simulink model "ITCG_PNG_3D_salvo_simulation2"  (R2023b)
settings: Solver=ode4  StartTime=0.0  StopTime=30  FixedStep=1/10  RelTol=1e-3
libraries: simulink x4, simulink_extras x4
(part 1 of 2)
settings Model: NumberOfSteps=10  PacingRate=5  Creator=Administrator  LastModifiedBy=Administrator
settings DebuggingCC: UnderSpecifiedDimensionMsg=warning

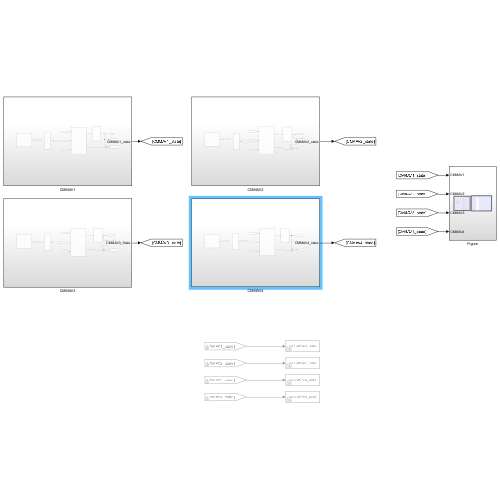
[thumbnail: Simulink's stored preview of the top-level diagram]
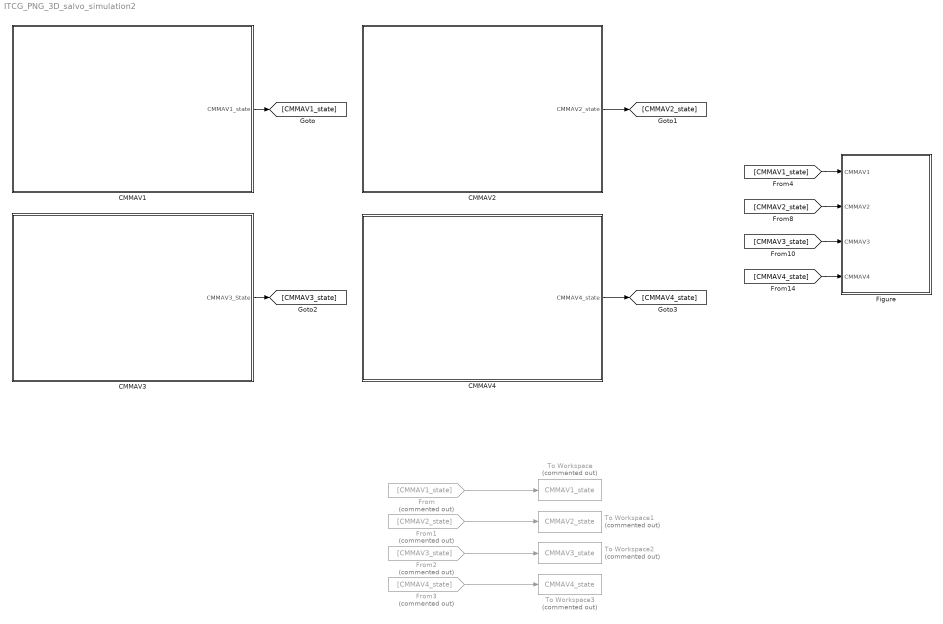
== system ITCG_PNG_3D_salvo_simulation2 ==
  CMMAV1 : Subsystem
  CMMAV2 : Subsystem
  CMMAV3 : Subsystem
  CMMAV4 : Subsystem
  Figure : Subsystem
  From : From  Commented=on  GotoTag=CMMAV1_state
  From1 : From  Commented=on  GotoTag=CMMAV2_state
  From2 : From  Commented=on  GotoTag=CMMAV3_state
  From3 : From  Commented=on  GotoTag=CMMAV4_state
  To Workspace : ToWorkspace  Commented=on  VariableName=CMMAV1_state  SaveFormat=Timeseries  SampleTime=-1
  To Workspace1 : ToWorkspace  Commented=on  VariableName=CMMAV2_state  SaveFormat=Timeseries  SampleTime=-1
  To Workspace2 : ToWorkspace  Commented=on  VariableName=CMMAV3_state  SaveFormat=Timeseries  SampleTime=-1
  To Workspace3 : ToWorkspace  Commented=on  VariableName=CMMAV4_state  SaveFormat=Timeseries  SampleTime=-1
  wires:
  CMMAV1/1(CMMAV1_state) -> [CMMAV1_state]
  CMMAV2/1(CMMAV2_state) -> [CMMAV2_state]
  CMMAV3/1(CMMAV3_State) -> [CMMAV3_state]
  CMMAV4/1(CMMAV4_state) -> [CMMAV4_state]
  From/1 -> To Workspace/1
  From1/1 -> To Workspace1/1
  From2/1 -> To Workspace2/1
  From3/1 -> To Workspace3/1
  [CMMAV2_state] -> Figure/2(CMMAV2)
  [CMMAV1_state] -> Figure/1(CMMAV1)
  [CMMAV3_state] -> Figure/3(CMMAV3)
  [CMMAV4_state] -> Figure/4(CMMAV4)

== system ITCG_PNG_3D_salvo_simulation2/CMMAV1 ==
  Guidance : Subsystem
  Mux : Mux  Inputs=2
  Parameter init : Subsystem
  Point Mass Model : Subsystem
  Target : Subsystem  TreatAsAtomicUnit=on
  To File : ToFile  Filename=CMMAV1_ITCG_PNG.mat
  CMMAV1_state : Outport
  wires:
  [Parameter] -> Guidance/3(Parameter)
  [Taregt_info] -> Guidance/2(Target_info)
  [CMMAV1_state] -> Guidance/1(CMMAV1_state)
  Guidance/1(CMMAV1_input) -> Point Mass Model/1(CMMAV1_input)
  Parameter init/1(Parameter) -> [Parameter]
  Guidance/2(CMMAV1_param) -> Mux/2
  Mux/1 -> To File/1
  Point Mass Model/1(CMMAV1_state) -> [CMMAV1_state], Mux/1, CMMAV1_state/1
  Target/1(Target_info) -> [Taregt_info]

== system ITCG_PNG_3D_salvo_simulation2/CMMAV2 ==
  CMMAV2 : Subsystem
  Guidance : Subsystem
  Mux : Mux  Inputs=2
  Parameter init : Subsystem
  Target : Subsystem  TreatAsAtomicUnit=on
  To File : ToFile  Filename=CMMAV2_ITCG_PNG.mat
  CMMAV2_state : Outport
  wires:
  [Parameter] -> Guidance/3(Parameter)
  Guidance/1(CMMAV2_input) -> CMMAV2/1(CMMAV2_input)
  [CMMAV2_state] -> Guidance/1(CMMAV2_state)
  Parameter init/1(Parameter) -> [Parameter]
  [Taregt_info] -> Guidance/2(Target_info)
  Guidance/2(CMMAV2_param) -> Mux/2
  Mux/1 -> To File/1
  CMMAV2/1(CMMAV2_state) -> [CMMAV2_state], Mux/1, CMMAV2_state/1
  Target/1(Target_info) -> [Taregt_info]

== system ITCG_PNG_3D_salvo_simulation2/CMMAV3 ==
  CMMAV3 : Subsystem
  Guidance : Subsystem
  Mux : Mux  Inputs=2
  Parameter init : Subsystem
  Target : Subsystem  TreatAsAtomicUnit=on
  To File : ToFile  Filename=CMMAV3_ITCG_PNG.mat
  CMMAV3_State : Outport
  wires:
  [Taregt_info] -> Guidance/2(Target_info)
  [Parameter] -> Guidance/3(Parameter)
  Parameter init/1(Parameter) -> [Parameter]
  Guidance/1(CMMAV3_input) -> CMMAV3/1(CMMAV3_input)
  [CMMAV3_state] -> Guidance/1(CMMAV3_state)
  Guidance/2(CMMAV1_param) -> Mux/2
  Mux/1 -> To File/1
  CMMAV3/1(CMMAV3_state) -> [CMMAV3_state], Mux/1, CMMAV3_State/1
  Target/1(Target_info) -> [Taregt_info]

== system ITCG_PNG_3D_salvo_simulation2/CMMAV4 ==
  CMMAV4 : Subsystem
  Guidance : Subsystem
  Mux : Mux  Inputs=2
  Parameter init : Subsystem
  Target : Subsystem  TreatAsAtomicUnit=on
  To File : ToFile  Filename=CMMAV4_ITCG_PNG.mat
  CMMAV4_state : Outport
  wires:
  [Taregt_info] -> Guidance/2(Target_info)
  Guidance/1(CMMAV4_input) -> CMMAV4/1(CMMAV4_input)
  [CMMAV4_state] -> Guidance/1(CMMAV4_state)
  [Parameter] -> Guidance/3(Parameter)
  Parameter init/1(Parameter) -> [Parameter]
  CMMAV4/1(CMMAV4_state) -> [CMMAV4_state], Mux/1, CMMAV4_state/1
  Mux/1 -> To File/1
  Guidance/2(CMMAV1_param) -> Mux/2
  Target/1(Target_info) -> [Taregt_info]

== system ITCG_PNG_3D_salvo_simulation2/Figure ==
  note: Figure
  note: Input parameter
  CMMAV1 : Inport
  CMMAV2 : Inport  Port=2
  CMMAV3 : Inport  Port=3
  CMMAV4 : Inport  Port=4
  Bus Selector{,1..3} (4 alike) : BusSelector  OutputSignals=Pos_M_m
  Demux{,1..3} (4 alike) : Demux  Outputs=3
  MATLAB Function : MATLAB Function  TreatAsAtomicUnit=on
  wires:
  Demux/2 -> [CMMAV1_y]
  Demux/1 -> [CMMAV1_x]
  Demux/3 -> [CMMAV1_z]
  [CMMAV1] -> Demux/1
  CMMAV1/1 -> Bus Selector/1
  CMMAV2/1 -> Bus Selector1/1
  CMMAV3/1 -> Bus Selector2/1
  CMMAV4/1 -> Bus Selector3/1
  Bus Selector/1 -> [CMMAV1]  "<Pos_M_m>"
  Bus Selector1/1 -> [CMMAV2]  "<Pos_M_m>"
  Bus Selector2/1 -> [CMMAV3]  "<Pos_M_m>"
  Bus Selector3/1 -> [CMMAV4]  "<Pos_M_m>"
  Demux1/1 -> [CMMAV2_x]
  Demux1/3 -> [CMMAV2_z]
  Demux1/2 -> [CMMAV2_y]
  [CMMAV2] -> Demux1/1
  Demux2/2 -> [CMMAV3_y]
  Demux2/1 -> [CMMAV3_x]
  Demux2/3 -> [CMMAV3_z]
  [CMMAV3] -> Demux2/1
  Demux3/2 -> [CMMAV4_y]
  Demux3/1 -> [CMMAV4_x]
  Demux3/3 -> [CMMAV4_z]
  [CMMAV4] -> Demux3/1
  [CMMAV1_x] -> MATLAB Function/1(CMMAV1_x)
  [CMMAV1_y] -> MATLAB Function/2(CMMAV1_y)
  [CMMAV1_z] -> MATLAB Function/3(CMMAV1_z)
  [CMMAV2_x] -> MATLAB Function/4(CMMAV2_x)
  [CMMAV2_y] -> MATLAB Function/5(CMMAV2_y)
  [CMMAV2_z] -> MATLAB Function/6(CMMAV2_z)
  [CMMAV3_x] -> MATLAB Function/7(CMMAV3_x)
  [CMMAV3_y] -> MATLAB Function/8(CMMAV3_y)
  [CMMAV3_z] -> MATLAB Function/9(CMMAV3_z)
  [CMMAV4_x] -> MATLAB Function/10(CMMAV4_x)
  [CMMAV4_y] -> MATLAB Function/11(CMMAV4_y)
  [CMMAV4_z] -> MATLAB Function/12(CMMAV4_z)

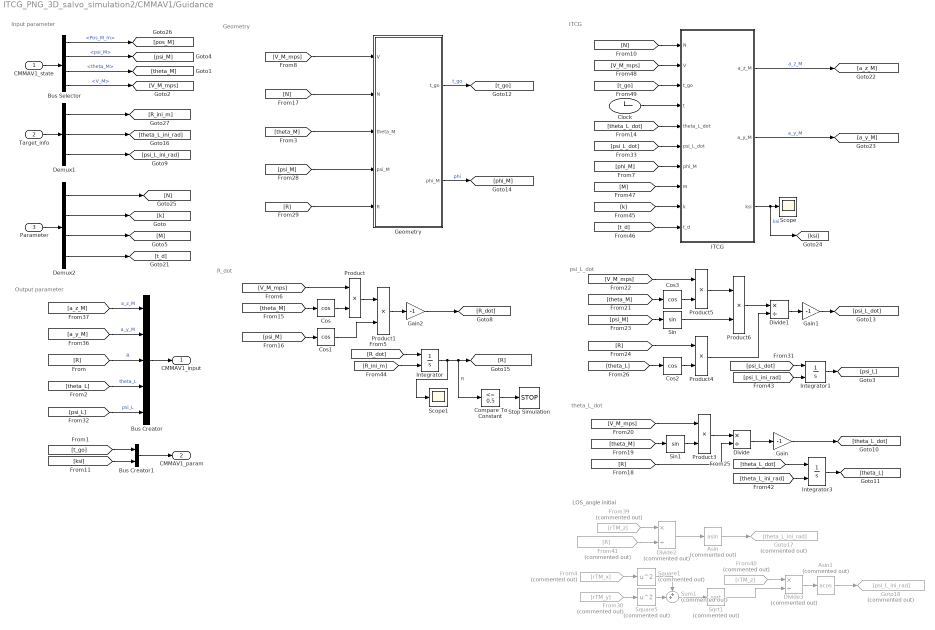
== system ITCG_PNG_3D_salvo_simulation2/CMMAV1/Guidance ==
  note: Input parameter
  note: ITCG
  note: R_dot
  note: psi_L_dot
  note: theta_L_dot
  note: LOS_angle initial
  note: Output parameter
  note: Geometry
  CMMAV1_state : Inport
  Target_info : Inport  Port=2
  Parameter : Inport  Port=3
  Asin : Trigonometry  Commented=on  Operator=asin
  Asin1 : Trigonometry  Commented=on  Operator=acos
  Bus Creator : BusCreator  Inputs=5
  Bus Creator1 : BusCreator  Inputs=2
  Bus Selector : BusSelector  OutputSignals=Pos_M_m,psi_M,theta_M,V_M
  Clock : Clock
  Compare To Constant : simulink/Logic and Bit Operations/Compare To Constant  relop=<=  const=0.5  OutDataTypeStr=boolean
  Cos{,1..3} (4 alike) : Trigonometry  Operator=cos
  Demux1 : Demux  Outputs=3
  Demux2 : Demux
  Divide : Product  Inputs=*/
  Divide1 : Product  Inputs=*/
  Divide2 : Product  Commented=on  Inputs=*/
  Divide3 : Product  Commented=on  Inputs=*/
  From30 : From  Commented=on  GotoTag=rTM_y
  From39 : From  Commented=on  GotoTag=rTM_z
  From4 : From  Commented=on  GotoTag=rTM_x
  From40 : From  Commented=on  GotoTag=rTM_z
  From41 : From  Commented=on  GotoTag=R
  Gain : Gain  Gain=-1
  Gain1 : Gain  Gain=-1
  Gain2 : Gain  Gain=-1
  Geometry : MATLAB Function  TreatAsAtomicUnit=on
  Goto17 : Goto  Commented=on  GotoTag=theta_L_ini_rad
  Goto18 : Goto  Commented=on  GotoTag=psi_L_ini_rad
  ITCG : MATLAB Function  TreatAsAtomicUnit=on
  Integrator : Integrator  InitialConditionSource=external  InitialCondition=sqrt(300^2+500^2+200^2)
  Integrator1 : Integrator  InitialConditionSource=external
  Integrator3 : Integrator  InitialConditionSource=external
  Product{,1,3..6} (6 alike) : Product
  Scope : Scope
  Scope1 : Scope
  Sin : Trigonometry
  Sin1 : Trigonometry
  Sqrt1 : Sqrt  Commented=on
  Square1 : Math  Commented=on  Operator=square
  Square5 : Math  Commented=on  Operator=square
  Stop Simulation : Stop
  Sum1 : Sum  Commented=on  Inputs=++|
  CMMAV1_input : Outport
  CMMAV1_param : Outport  Port=2
  wires:
  Product1/1 -> Gain2/1
  Gain2/1 -> [R_dot]
  [theta_L] -> Cos2/1
  [theta_L_dot] -> Integrator3/1
  Gain/1 -> [theta_L_dot]
  Product5/1 -> Product6/1
  Divide1/1 -> Gain1/1
  [V_M_mps] -> Product3/1
  [V_M_mps] -> Product5/1
  [theta_M] -> Sin1/1
  [R] -> Divide/2
  [theta_M] -> Cos3/1
  Divide/1 -> Gain/1
  [theta_M] -> Cos/1
  [R] -> Product4/1
  Product4/1 -> Divide1/2
  Integrator3/1 -> [theta_L]
  [psi_L_dot] -> Integrator1/1
  Sin1/1 -> Product3/2
  Product3/1 -> Divide/1
  [psi_M] -> Cos1/1
  Cos/1 -> Product/2
  Integrator1/1 -> [psi_L]
  Product6/1 -> Divide1/1
  [psi_M] -> Sin/1
  Compare To Constant/1 -> Stop Simulation/1
  [V_M_mps] -> Product/1
  Cos3/1 -> Product5/2
  Sin/1 -> Product6/2
  Integrator/1 -> Scope1/1, [R], Compare To Constant/1  "R"
  Product/1 -> Product1/1
  Cos2/1 -> Product4/2
  Cos1/1 -> Product1/2
  Gain1/1 -> [psi_L_dot]
  [R_dot] -> Integrator/1
  Divide3/1 -> Asin1/1
  Sum1/1 -> Sqrt1/1
  From30/1 -> Square5/1
  Square5/1 -> Sum1/2
  Square1/1 -> Sum1/1
  Asin/1 -> Goto17/1
  Sqrt1/1 -> Divide3/2
  From41/1 -> Divide2/2
  Asin1/1 -> Goto18/1
  From40/1 -> Divide3/1
  From39/1 -> Divide2/1
  From4/1 -> Square1/1
  Divide2/1 -> Asin/1
  CMMAV1_state/1 -> Bus Selector/1
  Target_info/1 -> Demux1/1
  Demux2/1 -> [N]
  Parameter/1 -> Demux2/1
  Bus Selector/1 -> [pos_M]  "<Pos_M_m>"
  Bus Selector/4 -> [V_M_mps]  "<V_M>"
  Demux1/2 -> [theta_L_ini_rad]
  Demux1/3 -> [psi_L_ini_rad]
  Demux1/1 -> [R_ini_m]
  [psi_L] -> Bus Creator/5  "psi_L"
  [theta_L] -> Bus Creator/4  "theta_L"
  Bus Creator/1 -> CMMAV1_input/1
  [a_y_M] -> Bus Creator/2  "a_y_M"
  [R] -> Bus Creator/3  "R"
  [a_z_M] -> Bus Creator/1  "a_z_M"
  [theta_L_ini_rad] -> Integrator3/2
  [psi_L_ini_rad] -> Integrator1/2
  [R_ini_m] -> Integrator/2
  Bus Selector/2 -> [psi_M]  "<psi_M>"
  Bus Selector/3 -> [theta_M]  "<theta_M>"
  Geometry/1(t_go) -> [t_go]  "t_go"
  [psi_M] -> Geometry/4(psi_M)
  Geometry/2(phi_M) -> [phi_M]  "phi"
  [V_M_mps] -> Geometry/1(V)
  [theta_M] -> Geometry/3(theta_M)
  [R] -> Geometry/5(R)
  [N] -> Geometry/2(N)
  [psi_L_dot] -> ITCG/6(psi_L_dot)
  Clock/1 -> ITCG/4(t)
  [t_go] -> ITCG/3(t_go)
  [N] -> ITCG/1(N)
  [M] -> ITCG/8(M)
  [k] -> ITCG/9(k)
  [t_d] -> ITCG/10(t_d)
  [phi_M] -> ITCG/7(phi_M)
  [theta_L_dot] -> ITCG/5(theta_L_dot)
  [V_M_mps] -> ITCG/2(V)
  Demux2/2 -> [k]
  Demux2/3 -> [M]
  Demux2/4 -> [t_d]
  ITCG/1(a_z_M) -> [a_z_M]  "a_z_M"
  ITCG/2(a_y_M) -> [a_y_M]  "a_y_M"
  ITCG/3(ksi) -> [ksi], Scope/1  "ksi"
  [t_go] -> Bus Creator1/1
  [ksi] -> Bus Creator1/2
  Bus Creator1/1 -> CMMAV1_param/1

== system ITCG_PNG_3D_salvo_simulation2/CMMAV1/Parameter init ==
  Constant : Constant  Value=3
  Constant1 : Constant  Value=2
  Constant2 : Constant  Value=10
  Constant3 : Constant  Value=30
  Mux : Mux
  Parameter : Outport
  wires:
  Mux/1 -> Parameter/1
  Constant3/1 -> Mux/4
  Constant2/1 -> Mux/3
  Constant1/1 -> Mux/2
  Constant/1 -> Mux/1

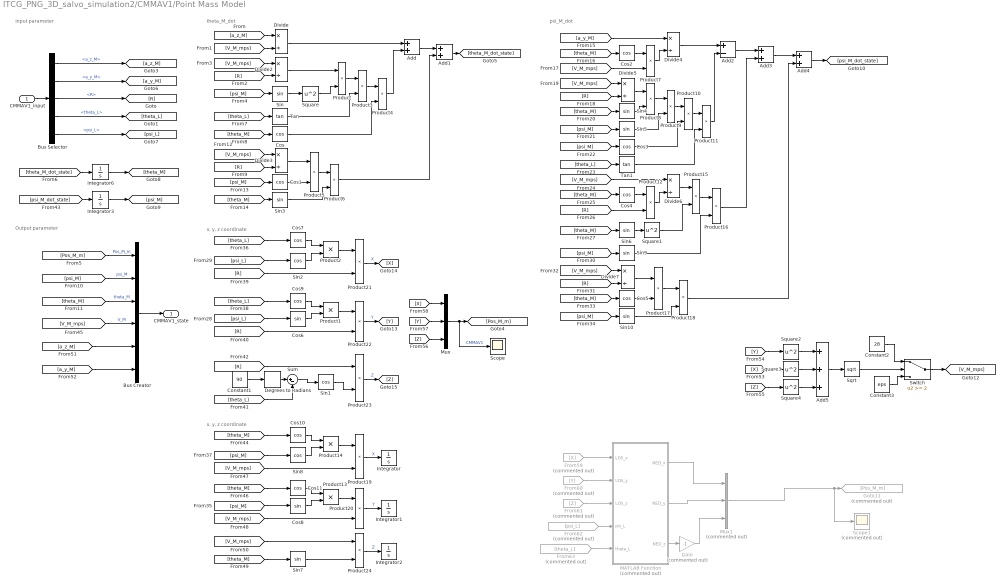
== system ITCG_PNG_3D_salvo_simulation2/CMMAV1/Point Mass Model ==
  note: Input parameter
  note: x, y, z coordinate
  note: theta_M_dot
  note: Output parameter
  note: psi_M_dot
  note: x, y, z coordinate
  CMMAV1_input : Inport
  Add{,1,3..4} (4 alike) : Sum
  Add2 : Sum  Inputs=+-
  Add5 : Sum  Inputs=+++
  Bus Creator : BusCreator  Inputs=6
  Bus Selector : BusSelector  OutputSignals=a_z_M,a_y_M,R,theta_L,psi_L
  Constant1 : Constant  Value=90
  Constant2 : Constant  Value=28
  Constant3 : Constant  Value=eps
  Cos{,1..5,7,9..11} (10 alike) : Trigonometry  Operator=cos
  Cos6 : Trigonometry
  Cos8 : Trigonometry
  Degrees to Radians : simulink_extras/Transformations/Degrees to Radians
  Divide{,2..7} (7 alike) : Product  Inputs=*/
  From59 : From  Commented=on  GotoTag=X
  From60 : From  Commented=on  GotoTag=Y
  From61 : From  Commented=on  GotoTag=Z
  From62 : From  Commented=on  GotoTag=psi_L
  From63 : From  Commented=on  GotoTag=theta_L
  Gain : Gain  Commented=on  Gain=-1
  Goto11 : Goto  Commented=on  GotoTag=Pos_M_m
  Integrator : Integrator
  Integrator1 : Integrator
  Integrator2 : Integrator
  Integrator3 : Integrator  InitialCondition=10*pi/180
  Integrator6 : Integrator  InitialCondition=10*pi/180
  MATLAB Function : MATLAB Function  Commented=on  TreatAsAtomicUnit=on
  Mux : Mux  Inputs=3
  Mux1 : Mux  Commented=on  Inputs=3
  Product{,1..24} (25 alike) : Product
  Scope : Scope
  Scope1 : Scope  Commented=on
  Sin{,3..7,9..10} (8 alike) : Trigonometry
  Sin1 : Trigonometry  Operator=cos
  Sin2 : Trigonometry  Operator=cos
  Sin8 : Trigonometry  Operator=cos
  Sqrt : Sqrt
  Square{,1..4} (5 alike) : Math  Operator=square
  Sum : Sum  Inputs=|+-
  Switch : Switch  Threshold=2  SaturateOnIntegerOverflow=off  InputSameDT=off
  Tan : Trigonometry  Operator=tan
  Tan1 : Trigonometry  Operator=tan
  CMMAV1_state : Outport
  wires:
  [theta_L] -> Tan1/1
  Product16/1 -> Add3/2
  Product9/1 -> Product10/1
  [psi_M] -> Bus Creator/2  "psi_M"
  Tan/1 -> Product3/2
  [psi_M_dot_state] -> Integrator3/1
  [psi_M] -> Sin9/1
  [theta_M] -> Cos/1
  Sin10/1 -> Product18/2
  [psi_M] -> Sin5/1
  Product17/1 -> Product18/1
  [psi_M] -> Sin10/1
  [theta_L] -> Cos9/1
  [V_M_mps] -> Divide/2
  Sin6/1 -> Square1/1
  Product15/1 -> Product16/1
  [V_M_mps] -> Bus Creator/4  "V_M"
  Cos5/1 -> Product17/2
  Sin/1 -> Square/1
  Add2/1 -> Add3/1
  Divide7/1 -> Product17/1
  [theta_M] -> Sin6/1
  [R] -> Divide7/2
  Sin3/1 -> Product6/2
  Add1/1 -> [theta_M_dot_state]
  Sin9/1 -> Product16/2
  Divide6/1 -> Product15/1
  Square1/1 -> Product15/2
  [R] -> Divide3/2
  [a_z_M] -> Divide/1
  [theta_M] -> Cos5/1
  Add3/1 -> Add4/1
  Product12/1 -> Divide6/2
  Product8/1 -> Product9/1
  [a_y_M] -> Divide4/1
  [psi_M] -> Cos3/1
  Product10/1 -> Product11/1
  Product3/1 -> Product4/1
  Divide4/1 -> Add2/1
  Cos3/1 -> Product10/2
  Product11/1 -> Add2/2
  [R] -> Product12/2
  [V_M_mps] -> Divide5/1
  Cos/1 -> Product4/2
  Product5/1 -> Product6/1
  Product6/1 -> Add1/2
  Divide3/1 -> Product5/1
  Cos1/1 -> Product5/2
  Square/1 -> Product/2
  [psi_M] -> Cos1/1
  [V_M_mps] -> Product7/2
  [R] -> Divide2/2
  Cos6/1 -> Product1/2
  [V_M_mps] -> Divide2/1
  [psi_M] -> Sin/1
  Bus Selector/2 -> [a_y_M]  "<a_y_M>"
  [theta_M] -> Sin4/1
  Tan1/1 -> Product11/2
  Integrator6/1 -> [theta_M]
  [theta_M] -> Sin3/1
  [psi_L] -> Cos6/1
  Add/1 -> Add1/1
  Bus Selector/5 -> [psi_L]  "<psi_L>"
  [R] -> Divide5/2
  Product21/1 -> [X]  "X"
  [V_M_mps] -> Divide6/1
  Product1/1 -> Product22/1
  Integrator3/1 -> [psi_M]
  Product/1 -> Product3/1
  Sin2/1 -> Product2/2
  Bus Selector/1 -> [a_z_M]  "<a_z_M>"
  Add4/1 -> [psi_M_dot_state]
  [V_M_mps] -> Divide7/1
  Cos2/1 -> Product7/1
  Mux/1 -> [Pos_M_m], Scope/1  "CMMAV1"
  Bus Selector/3 -> [R]  "<R>"
  [theta_M] -> Bus Creator/3  "theta_M"
  [psi_L] -> Sin2/1
  Divide2/1 -> Product/1
  [theta_M] -> Cos2/1
  Sin4/1 -> Product8/2
  [theta_L] -> Tan/1
  Cos4/1 -> Product12/1
  Product2/1 -> Product21/1
  [theta_M] -> Cos4/1
  Cos9/1 -> Product1/1
  [V_M_mps] -> Divide3/1
  Sin5/1 -> Product9/2
  [theta_L] -> Cos7/1
  Product4/1 -> Add/2
  Product18/1 -> Add4/2
  Product7/1 -> Divide4/2
  Divide5/1 -> Product8/1
  Divide/1 -> Add/1
  Cos7/1 -> Product2/1
  [theta_M_dot_state] -> Integrator6/1
  Product22/1 -> [Y]  "Y"
  [V_M_mps] -> Product24/1
  Sin7/1 -> Product24/2
  [V_M_mps] -> Product20/2
  [theta_M] -> Cos11/1
  [psi_M] -> Sin8/1
  [theta_M] -> Sin7/1
  Sin8/1 -> Product14/2
  Product14/1 -> Product19/1
  Product19/1 -> Integrator/1  "X"
  Product13/1 -> Product20/1
  Product24/1 -> Integrator2/1  "Z"
  [psi_M] -> Cos8/1
  [V_M_mps] -> Product19/2
  [theta_M] -> Cos10/1
  Cos11/1 -> Product13/1
  Cos8/1 -> Product13/2
  Product20/1 -> Integrator1/1  "Y"
  Cos10/1 -> Product14/1
  [R] -> Product21/2
  [R] -> Product22/2
  [R] -> Product23/1
  Constant1/1 -> Degrees to Radians/1
  Degrees to Radians/1 -> Sum/1
  Sin1/1 -> Product23/2
  [theta_L] -> Sum/2
  Sum/1 -> Sin1/1
  CMMAV1_input/1 -> Bus Selector/1
  [Pos_M_m] -> Bus Creator/1  "Pos_M_m"
  Bus Creator/1 -> CMMAV1_state/1
  Bus Selector/4 -> [theta_L]  "<theta_L>"
  [a_z_M] -> Bus Creator/5
  [a_y_M] -> Bus Creator/6
  Constant3/1 -> Switch/3
  Switch/1 -> [V_M_mps]
  Sqrt/1 -> Switch/2
  Add5/1 -> Sqrt/1
  Square2/1 -> Add5/1
  [Y] -> Square2/1
  Constant2/1 -> Switch/1
  [X] -> Square3/1
  Square3/1 -> Add5/2
  Product23/1 -> [Z]  "Z"
  [Z] -> Square4/1
  [X] -> Mux/1
  [Y] -> Mux/2
  [Z] -> Mux/3
  Square4/1 -> Add5/3
  From59/1 -> MATLAB Function/1(LOS_x)
  From60/1 -> MATLAB Function/2(LOS_y)
  From61/1 -> MATLAB Function/3(LOS_z)
  From62/1 -> MATLAB Function/4(psi_L)
  From63/1 -> MATLAB Function/5(theta_L)
  MATLAB Function/2(NED_y) -> Mux1/2
  MATLAB Function/1(NED_x) -> Mux1/1
  MATLAB Function/3(NED_z) -> Gain/1
  Gain/1 -> Mux1/3
  Mux1/1 -> Scope1/1, Goto11/1

== system ITCG_PNG_3D_salvo_simulation2/CMMAV1/Target ==
  note: LOS_angle initial
  note: Target position
  note: Target parameter
  note: Output parameter
  note: R_initial
  note: Output parameter
  Add : Sum
  Add1 : Sum
  Add2 : Sum
  Asin : Trigonometry  Operator=asin
  Asin1 : Trigonometry  Operator=acos
  Demux : Demux  Outputs=3
  Demux1 : Demux  Outputs=3
  Divide : Product  Inputs=*/
  Divide1 : Product  Inputs=*/
  Integrator : Integrator
  Integrator1 : Integrator
  Integrator2 : Integrator
  Mux : Mux  Inputs=3
  Mux1 : Mux  Inputs=3
  Scope : Scope
  Sqrt : Sqrt
  Sqrt1 : Sqrt
  Square{1..5} (5 alike) : Math  Operator=square
  Sum : Sum  Inputs=+++
  Sum1 : Sum  Inputs=++|
  Target Position : Constant  Value=[300;500;300]  VectorParams1D=off
  Target Velocity : Constant  Value=[0;0;0]  VectorParams1D=off
  Target_info : Outport
  wires:
  [psi_L_ini_rad] -> Mux/3
  Asin/1 -> [theta_L_ini_rad]
  [rT_ini_z_m] -> Mux1/3
  [rM_z] -> Add2/1
  Demux/3 -> [vT_z]
  [vT_z] -> Integrator2/1
  Demux/2 -> [vT_y]
  [rT_ini_x_m] -> Mux1/1
  Add1/1 -> [rT_ini_y_m]  "Y"
  Square2/1 -> Sum/1
  [vT_x] -> Integrator/1
  Mux1/1 -> [Pos_T_m]
  Square3/1 -> Sum/2
  Add2/1 -> [rT_ini_z_m]  "Z"
  Integrator/1 -> [vT_xt]
  Sum/1 -> Sqrt/1
  Demux1/3 -> [rM_z]
  [rT_ini_y_m] -> Mux1/2
  Integrator1/1 -> [vT_yt]
  Demux/1 -> [vT_x]
  Demux1/1 -> [rM_x]
  Target Velocity/1 -> Demux/1
  Demux1/2 -> [rM_y]
  Add/1 -> [rT_ini_x_m]  "X"
  [vT_yt] -> Add1/2
  Divide1/1 -> Asin1/1
  [rM_x] -> Add/1
  [vT_zt] -> Add2/2
  Sum1/1 -> Sqrt1/1
  [rT_ini_x_m] -> Square1/1
  Square1/1 -> Sum1/1
  Square5/1 -> Sum1/2
  [rT_ini_y_m] -> Square5/1
  [vT_y] -> Integrator1/1
  [rM_y] -> Add1/1
  [rT_ini_z_m] -> Divide/1
  [R_ini_m] -> Mux/1
  Sqrt/1 -> Scope/1, [R_ini_m]
  [R_ini_m] -> Divide/2
  [rT_ini_z_m] -> Square4/1
  Sqrt1/1 -> Divide1/2
  [vT_xt] -> Add/2
  Divide/1 -> Asin/1
  Integrator2/1 -> [vT_zt]
  Square4/1 -> Sum/3
  [rT_ini_x_m] -> Divide1/1
  [theta_L_ini_rad] -> Mux/2
  Asin1/1 -> [psi_L_ini_rad]
  Mux/1 -> Target_info/1
  Target Position/1 -> Demux1/1
  [rT_ini_y_m] -> Square3/1
  [rT_ini_x_m] -> Square2/1

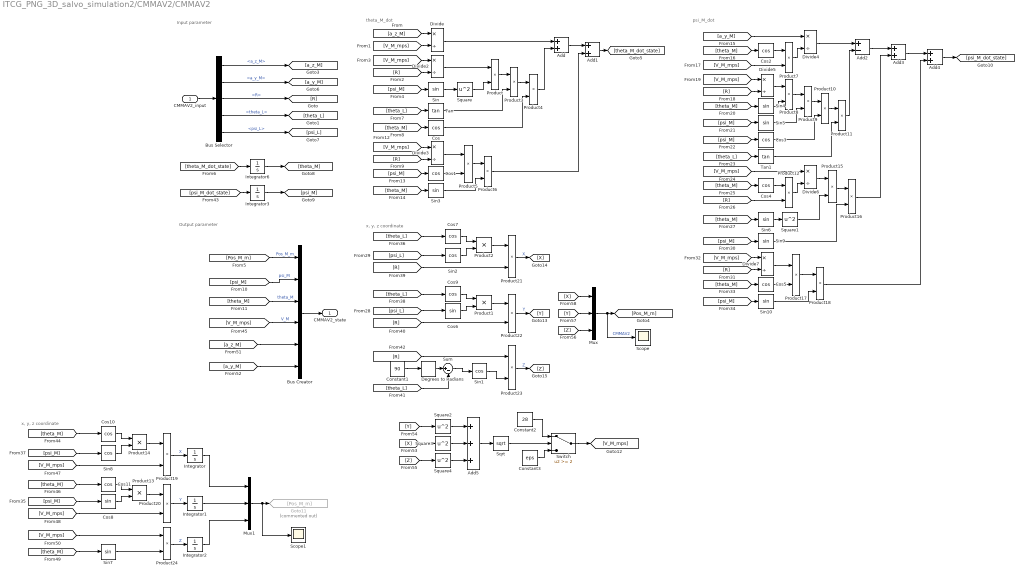
== system ITCG_PNG_3D_salvo_simulation2/CMMAV2/CMMAV2 ==
  note: theta_M_dot
  note: psi_M_dot
  note: x, y, z coordinate
  note: Input parameter
  note: Output parameter
  note: x, y, z coordinate
  CMMAV2_input : Inport
  Add{,1,3..4} (4 alike) : Sum
  Add2 : Sum  Inputs=+-
  Add5 : Sum  Inputs=+++
  Bus Creator : BusCreator  Inputs=6
  Bus Selector : BusSelector  OutputSignals=a_z_M,a_y_M,R,theta_L,psi_L
  Constant1 : Constant  Value=90
  Constant2 : Constant  Value=28
  Constant3 : Constant  Value=eps
  Cos{,1..5,7,9..11} (10 alike) : Trigonometry  Operator=cos
  Cos6 : Trigonometry
  Cos8 : Trigonometry
  Degrees to Radians : simulink_extras/Transformations/Degrees to Radians
  Divide{,2..7} (7 alike) : Product  Inputs=*/
  Goto11 : Goto  Commented=on  GotoTag=Pos_M_m
  Integrator : Integrator
  Integrator1 : Integrator
  Integrator2 : Integrator
  Integrator3 : Integrator  InitialCondition=10*pi/180
  Integrator6 : Integrator  InitialCondition=10*pi/180
  Mux : Mux  Inputs=3
  Mux1 : Mux  Inputs=3
  Product{,1..24} (25 alike) : Product
  Scope : Scope
  Scope1 : Scope
  Sin{,3..7,9..10} (8 alike) : Trigonometry
  Sin1 : Trigonometry  Operator=cos
  Sin2 : Trigonometry  Operator=cos
  Sin8 : Trigonometry  Operator=cos
  Sqrt : Sqrt
  Square{,1..4} (5 alike) : Math  Operator=square
  Sum : Sum  Inputs=|+-
  Switch : Switch  Threshold=2  SaturateOnIntegerOverflow=off  InputSameDT=off
  Tan : Trigonometry  Operator=tan
  Tan1 : Trigonometry  Operator=tan
  CMMAV2_state : Outport
  wires:
  [theta_L] -> Tan1/1
  Product16/1 -> Add3/2
  Product9/1 -> Product10/1
  Tan/1 -> Product3/2
  [psi_M] -> Sin9/1
  [theta_M] -> Cos/1
  Sin10/1 -> Product18/2
  [psi_M] -> Sin5/1
  Product17/1 -> Product18/1
  [psi_M] -> Sin10/1
  [V_M_mps] -> Divide/2
  Sin6/1 -> Square1/1
  Product15/1 -> Product16/1
  Cos5/1 -> Product17/2
  Sin/1 -> Square/1
  Add2/1 -> Add3/1
  Divide7/1 -> Product17/1
  [theta_M] -> Sin6/1
  [R] -> Divide7/2
  Sin3/1 -> Product6/2
  Add1/1 -> [theta_M_dot_state]
  Sin9/1 -> Product16/2
  Divide6/1 -> Product15/1
  Square1/1 -> Product15/2
  [R] -> Divide3/2
  [a_z_M] -> Divide/1
  [theta_M] -> Cos5/1
  Add3/1 -> Add4/1
  Product12/1 -> Divide6/2
  Product8/1 -> Product9/1
  [a_y_M] -> Divide4/1
  [psi_M] -> Cos3/1
  Product10/1 -> Product11/1
  Product3/1 -> Product4/1
  Divide4/1 -> Add2/1
  Cos3/1 -> Product10/2
  Product11/1 -> Add2/2
  [R] -> Product12/2
  [V_M_mps] -> Divide5/1
  Cos/1 -> Product4/2
  Product5/1 -> Product6/1
  Product6/1 -> Add1/2
  Divide3/1 -> Product5/1
  Cos1/1 -> Product5/2
  Square/1 -> Product/2
  [psi_M] -> Cos1/1
  [V_M_mps] -> Product7/2
  [R] -> Divide2/2
  [V_M_mps] -> Divide2/1
  [psi_M] -> Sin/1
  [theta_M] -> Sin4/1
  Tan1/1 -> Product11/2
  [theta_M] -> Sin3/1
  Add/1 -> Add1/1
  [R] -> Divide5/2
  [V_M_mps] -> Divide6/1
  Product/1 -> Product3/1
  Add4/1 -> [psi_M_dot_state]
  [V_M_mps] -> Divide7/1
  Cos2/1 -> Product7/1
  Divide2/1 -> Product/1
  [theta_M] -> Cos2/1
  Sin4/1 -> Product8/2
  [theta_L] -> Tan/1
  Cos4/1 -> Product12/1
  [theta_M] -> Cos4/1
  [V_M_mps] -> Divide3/1
  Sin5/1 -> Product9/2
  Product4/1 -> Add/2
  Product18/1 -> Add4/2
  Product7/1 -> Divide4/2
  Divide5/1 -> Product8/1
  Divide/1 -> Add/1
  [V_M_mps] -> Product24/1
  Sin7/1 -> Product24/2
  [V_M_mps] -> Product20/2
  [theta_M] -> Cos11/1
  [psi_M] -> Sin8/1
  Mux1/1 -> Scope1/1, Goto11/1
  [theta_M] -> Sin7/1
  Sin8/1 -> Product14/2
  Product14/1 -> Product19/1
  Product19/1 -> Integrator/1  "X"
  Product13/1 -> Product20/1
  Product24/1 -> Integrator2/1  "Z"
  [psi_M] -> Cos8/1
  [V_M_mps] -> Product19/2
  [theta_M] -> Cos10/1
  Cos11/1 -> Product13/1
  Cos8/1 -> Product13/2
  Product20/1 -> Integrator1/1  "Y"
  Cos10/1 -> Product14/1
  Integrator/1 -> Mux1/1
  Integrator1/1 -> Mux1/2
  Integrator2/1 -> Mux1/3
  Integrator3/1 -> [psi_M]
  [theta_M_dot_state] -> Integrator6/1
  [psi_M_dot_state] -> Integrator3/1
  Integrator6/1 -> [theta_M]
  Bus Selector/2 -> [a_y_M]  "<a_y_M>"
  Bus Selector/1 -> [a_z_M]  "<a_z_M>"
  Bus Selector/4 -> [theta_L]  "<theta_L>"
  Bus Selector/3 -> [R]  "<R>"
  Bus Selector/5 -> [psi_L]  "<psi_L>"
  CMMAV2_input/1 -> Bus Selector/1
  [a_y_M] -> Bus Creator/6
  [Pos_M_m] -> Bus Creator/1  "Pos_M_m"
  [a_z_M] -> Bus Creator/5
  [theta_M] -> Bus Creator/3  "theta_M"
  [psi_M] -> Bus Creator/2  "psi_M"
  Bus Creator/1 -> CMMAV2_state/1
  [V_M_mps] -> Bus Creator/4  "V_M"
  [X] -> Mux/1
  Constant2/1 -> Switch/1
  Sqrt/1 -> Switch/2
  Constant3/1 -> Switch/3
  [Z] -> Square4/1
  Switch/1 -> [V_M_mps]
  Square2/1 -> Add5/1
  Square4/1 -> Add5/3
  Product23/1 -> [Z]  "Z"
  [R] -> Product21/2
  [R] -> Product22/2
  Square3/1 -> Add5/2
  Sum/1 -> Sin1/1
  [theta_L] -> Sum/2
  Add5/1 -> Sqrt/1
  [psi_L] -> Sin2/1
  Degrees to Radians/1 -> Sum/1
  Mux/1 -> [Pos_M_m], Scope/1  "CMMAV2"
  [R] -> Product23/1
  Cos7/1 -> Product2/1
  Sin1/1 -> Product23/2
  [X] -> Square3/1
  [theta_L] -> Cos7/1
  Product1/1 -> Product22/1
  Product2/1 -> Product21/1
  Constant1/1 -> Degrees to Radians/1
  [Z] -> Mux/3
  Sin2/1 -> Product2/2
  Product21/1 -> [X]  "X"
  [Y] -> Mux/2
  [psi_L] -> Cos6/1
  [theta_L] -> Cos9/1
  [Y] -> Square2/1
  Cos9/1 -> Product1/1
  Cos6/1 -> Product1/2
  Product22/1 -> [Y]  "Y"

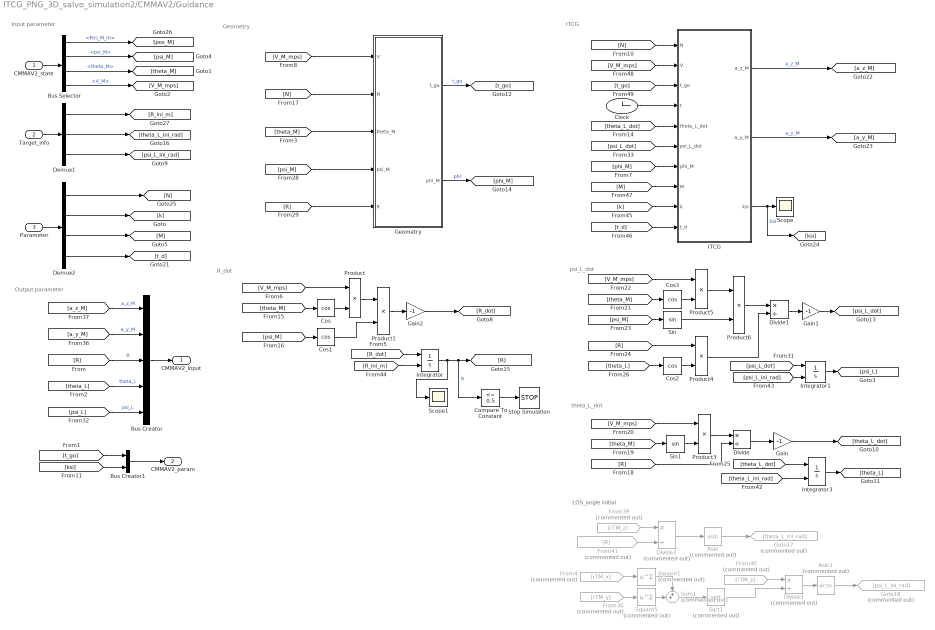
== system ITCG_PNG_3D_salvo_simulation2/CMMAV2/Guidance ==
  note: Input parameter
  note: R_dot
  note: psi_L_dot
  note: theta_L_dot
  note: LOS_angle initial
  note: Output parameter
  note: Geometry
  note: ITCG
  CMMAV2_state : Inport
  Target_info : Inport  Port=2
  Parameter : Inport  Port=3
  Asin : Trigonometry  Commented=on  Operator=asin
  Asin1 : Trigonometry  Commented=on  Operator=acos
  Bus Creator : BusCreator  Inputs=5
  Bus Creator1 : BusCreator  Inputs=2
  Bus Selector : BusSelector  OutputSignals=Pos_M_m,psi_M,theta_M,V_M
  Clock : Clock
  Compare To Constant : simulink/Logic and Bit Operations/Compare To Constant  relop=<=  const=0.5  OutDataTypeStr=boolean
  Cos{,1..3} (4 alike) : Trigonometry  Operator=cos
  Demux1 : Demux  Outputs=3
  Demux2 : Demux
  Divide : Product  Inputs=*/
  Divide1 : Product  Inputs=*/
  Divide2 : Product  Commented=on  Inputs=*/
  Divide3 : Product  Commented=on  Inputs=*/
  From30 : From  Commented=on  GotoTag=rTM_y
  From39 : From  Commented=on  GotoTag=rTM_z
  From4 : From  Commented=on  GotoTag=rTM_x
  From40 : From  Commented=on  GotoTag=rTM_z
  From41 : From  Commented=on  GotoTag=R
  Gain : Gain  Gain=-1
  Gain1 : Gain  Gain=-1
  Gain2 : Gain  Gain=-1
  Geometry : MATLAB Function  TreatAsAtomicUnit=on
  Goto17 : Goto  Commented=on  GotoTag=theta_L_ini_rad
  Goto18 : Goto  Commented=on  GotoTag=psi_L_ini_rad
  ITCG : MATLAB Function  TreatAsAtomicUnit=on
  Integrator : Integrator  InitialConditionSource=external  InitialCondition=sqrt(300^2+500^2+200^2)
  Integrator1 : Integrator  InitialConditionSource=external
  Integrator3 : Integrator  InitialConditionSource=external
  Product{,1,3..6} (6 alike) : Product
  Scope : Scope
  Scope1 : Scope
  Sin : Trigonometry
  Sin1 : Trigonometry
  Sqrt1 : Sqrt  Commented=on
  Square1 : Math  Commented=on  Operator=square
  Square5 : Math  Commented=on  Operator=square
  Stop Simulation : Stop
  Sum1 : Sum  Commented=on  Inputs=++|
  CMMAV2_input : Outport
  CMMAV2_param : Outport  Port=2
  wires:
  Product1/1 -> Gain2/1
  Gain2/1 -> [R_dot]
  [theta_L] -> Cos2/1
  [theta_L_dot] -> Integrator3/1
  Gain/1 -> [theta_L_dot]
  Product5/1 -> Product6/1
  Divide1/1 -> Gain1/1
  [V_M_mps] -> Product3/1
  [V_M_mps] -> Product5/1
  [theta_M] -> Sin1/1
  [R] -> Divide/2
  [theta_M] -> Cos3/1
  Divide/1 -> Gain/1
  [theta_M] -> Cos/1
  [R] -> Product4/1
  Product4/1 -> Divide1/2
  Integrator3/1 -> [theta_L]
  [psi_L_dot] -> Integrator1/1
  Sin1/1 -> Product3/2
  Product3/1 -> Divide/1
  [psi_M] -> Cos1/1
  Cos/1 -> Product/2
  Integrator1/1 -> [psi_L]
  Product6/1 -> Divide1/1
  [psi_M] -> Sin/1
  Compare To Constant/1 -> Stop Simulation/1
  [V_M_mps] -> Product/1
  Cos3/1 -> Product5/2
  Sin/1 -> Product6/2
  Integrator/1 -> Scope1/1, [R], Compare To Constant/1  "R"
  Product/1 -> Product1/1
  Cos2/1 -> Product4/2
  Cos1/1 -> Product1/2
  Gain1/1 -> [psi_L_dot]
  [R_dot] -> Integrator/1
  Divide3/1 -> Asin1/1
  Sum1/1 -> Sqrt1/1
  From30/1 -> Square5/1
  Square5/1 -> Sum1/2
  Square1/1 -> Sum1/1
  Asin/1 -> Goto17/1
  Sqrt1/1 -> Divide3/2
  From41/1 -> Divide2/2
  Asin1/1 -> Goto18/1
  From40/1 -> Divide3/1
  From39/1 -> Divide2/1
  From4/1 -> Square1/1
  Divide2/1 -> Asin/1
  CMMAV2_state/1 -> Bus Selector/1
  Target_info/1 -> Demux1/1
  Demux2/1 -> [N]
  Parameter/1 -> Demux2/1
  Bus Selector/1 -> [pos_M]  "<Pos_M_m>"
  Bus Selector/4 -> [V_M_mps]  "<V_M>"
  Demux1/2 -> [theta_L_ini_rad]
  Demux1/3 -> [psi_L_ini_rad]
  Demux1/1 -> [R_ini_m]
  [psi_L] -> Bus Creator/5  "psi_L"
  [theta_L] -> Bus Creator/4  "theta_L"
  Bus Creator/1 -> CMMAV2_input/1
  [a_y_M] -> Bus Creator/2  "a_y_M"
  [R] -> Bus Creator/3  "R"
  [a_z_M] -> Bus Creator/1  "a_z_M"
  [theta_L_ini_rad] -> Integrator3/2
  [psi_L_ini_rad] -> Integrator1/2
  [R_ini_m] -> Integrator/2
  Bus Selector/2 -> [psi_M]  "<psi_M>"
  Bus Selector/3 -> [theta_M]  "<theta_M>"
  Geometry/1(t_go) -> [t_go]  "t_go"
  [psi_M] -> Geometry/4(psi_M)
  Geometry/2(phi_M) -> [phi_M]  "phi"
  [V_M_mps] -> Geometry/1(V)
  [theta_M] -> Geometry/3(theta_M)
  [R] -> Geometry/5(R)
  [N] -> Geometry/2(N)
  Demux2/2 -> [k]
  Demux2/3 -> [M]
  Demux2/4 -> [t_d]
  [ksi] -> Bus Creator1/2
  [t_go] -> Bus Creator1/1
  Bus Creator1/1 -> CMMAV2_param/1
  ITCG/3(ksi) -> [ksi], Scope/1  "ksi"
  [t_d] -> ITCG/10(t_d)
  ITCG/1(a_z_M) -> [a_z_M]  "a_z_M"
  ITCG/2(a_y_M) -> [a_y_M]  "a_y_M"
  [theta_L_dot] -> ITCG/5(theta_L_dot)
  [phi_M] -> ITCG/7(phi_M)
  [t_go] -> ITCG/3(t_go)
  [N] -> ITCG/1(N)
  [M] -> ITCG/8(M)
  Clock/1 -> ITCG/4(t)
  [V_M_mps] -> ITCG/2(V)
  [k] -> ITCG/9(k)
  [psi_L_dot] -> ITCG/6(psi_L_dot)

== system ITCG_PNG_3D_salvo_simulation2/CMMAV2/Parameter init ==
  Constant : Constant  Value=3
  Constant1 : Constant  Value=2
  Constant2 : Constant  Value=10
  Constant3 : Constant  Value=30
  Mux : Mux
  Parameter : Outport
  wires:
  Mux/1 -> Parameter/1
  Constant3/1 -> Mux/4
  Constant2/1 -> Mux/3
  Constant1/1 -> Mux/2
  Constant/1 -> Mux/1

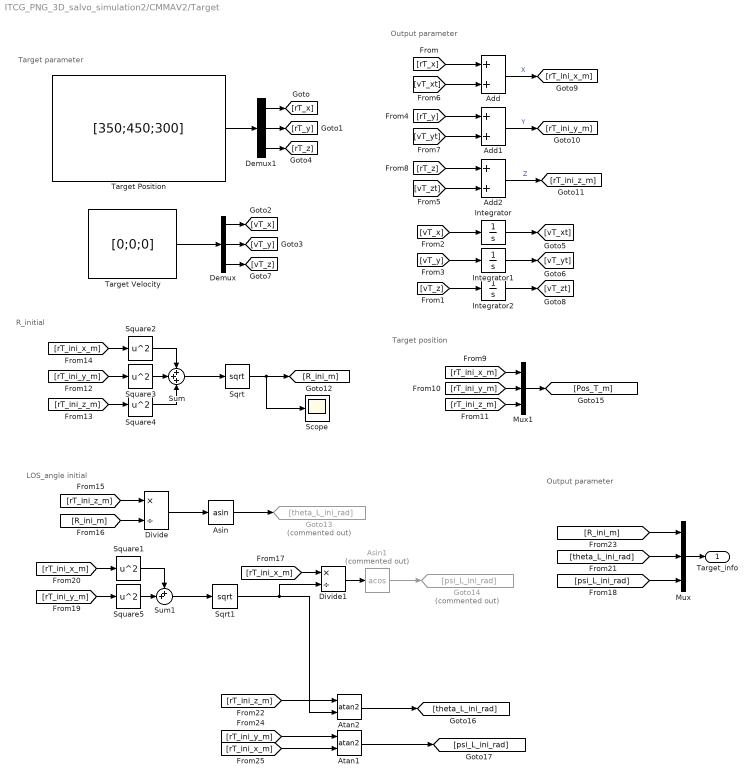
== system ITCG_PNG_3D_salvo_simulation2/CMMAV2/Target ==
  note: LOS_angle initial
  note: Target position
  note: Target parameter
  note: Output parameter
  note: R_initial
  note: Output parameter
  Add : Sum
  Add1 : Sum
  Add2 : Sum
  Asin : Trigonometry  Operator=asin
  Asin1 : Trigonometry  Commented=on  Operator=acos
  Atan1 : Trigonometry  Operator=atan2
  Atan2 : Trigonometry  Operator=atan2
  Demux : Demux  Outputs=3
  Demux1 : Demux  Outputs=3
  Divide : Product  Inputs=*/
  Divide1 : Product  Inputs=*/
  Goto13 : Goto  Commented=on  GotoTag=theta_L_ini_rad
  Goto14 : Goto  Commented=on  GotoTag=psi_L_ini_rad
  Integrator : Integrator
  Integrator1 : Integrator
  Integrator2 : Integrator
  Mux : Mux  Inputs=3
  Mux1 : Mux  Inputs=3
  Scope : Scope
  Sqrt : Sqrt
  Sqrt1 : Sqrt
  Square{1..5} (5 alike) : Math  Operator=square
  Sum : Sum  Inputs=+++
  Sum1 : Sum  Inputs=++|
  Target Position : Constant  Value=[350;450;300]  VectorParams1D=off
  Target Velocity : Constant  Value=[0;0;0]  VectorParams1D=off
  Target_info : Outport
  wires:
  [psi_L_ini_rad] -> Mux/3
  Asin/1 -> Goto13/1
  [rT_ini_z_m] -> Mux1/3
  [rT_z] -> Add2/1
  Demux/3 -> [vT_z]
  [vT_z] -> Integrator2/1
  Demux/2 -> [vT_y]
  [rT_ini_x_m] -> Mux1/1
  Add1/1 -> [rT_ini_y_m]  "Y"
  Square2/1 -> Sum/1
  [vT_x] -> Integrator/1
  Mux1/1 -> [Pos_T_m]
  Square3/1 -> Sum/2
  Add2/1 -> [rT_ini_z_m]  "Z"
  Target Position/1 -> Demux1/1
  Integrator/1 -> [vT_xt]
  Sum/1 -> Sqrt/1
  Demux1/3 -> [rT_z]
  [rT_ini_y_m] -> Mux1/2
  Integrator1/1 -> [vT_yt]
  Demux/1 -> [vT_x]
  Demux1/1 -> [rT_x]
  Target Velocity/1 -> Demux/1
  Demux1/2 -> [rT_y]
  Add/1 -> [rT_ini_x_m]  "X"
  [vT_yt] -> Add1/2
  Divide1/1 -> Asin1/1
  [rT_x] -> Add/1
  [vT_zt] -> Add2/2
  Sum1/1 -> Sqrt1/1
  [rT_ini_x_m] -> Square1/1
  Square1/1 -> Sum1/1
  Square5/1 -> Sum1/2
  [rT_ini_y_m] -> Square5/1
  [vT_y] -> Integrator1/1
  [rT_y] -> Add1/1
  [rT_ini_x_m] -> Square2/1
  [rT_ini_z_m] -> Divide/1
  [R_ini_m] -> Mux/1
  Sqrt/1 -> Scope/1, [R_ini_m]
  [R_ini_m] -> Divide/2
  [rT_ini_z_m] -> Square4/1
  [rT_ini_y_m] -> Square3/1
  [vT_xt] -> Add/2
  Divide/1 -> Asin/1
  Integrator2/1 -> [vT_zt]
  Square4/1 -> Sum/3
  [rT_ini_x_m] -> Divide1/1
  [theta_L_ini_rad] -> Mux/2
  Asin1/1 -> Goto14/1
  Mux/1 -> Target_info/1
  Sqrt1/1 -> Atan2/2, Divide1/2
  [rT_ini_z_m] -> Atan2/1
  Atan2/1 -> [theta_L_ini_rad]
  [rT_ini_x_m] -> Atan1/2
  [rT_ini_y_m] -> Atan1/1
  Atan1/1 -> [psi_L_ini_rad]

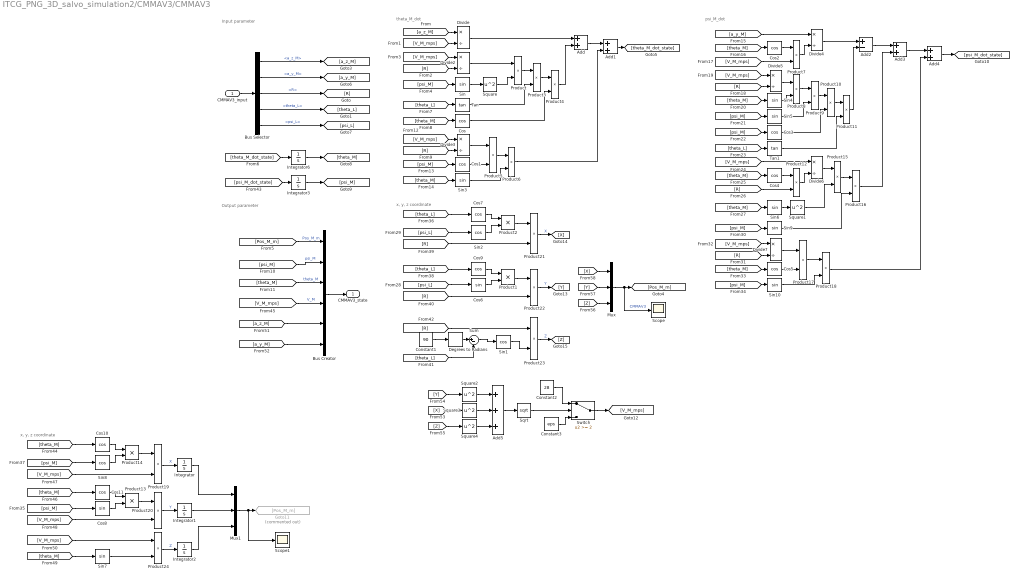
== system ITCG_PNG_3D_salvo_simulation2/CMMAV3/CMMAV3 ==
  note: theta_M_dot
  note: psi_M_dot
  note: x, y, z coordinate
  note: Input parameter
  note: Output parameter
  note: x, y, z coordinate
  CMMAV3_input : Inport
  Add{,1,3..4} (4 alike) : Sum
  Add2 : Sum  Inputs=+-
  Add5 : Sum  Inputs=+++
  Bus Creator : BusCreator  Inputs=6
  Bus Selector : BusSelector  OutputSignals=a_z_M,a_y_M,R,theta_L,psi_L
  Constant1 : Constant  Value=90
  Constant2 : Constant  Value=28
  Constant3 : Constant  Value=eps
  Cos{,1..5,7,9..11} (10 alike) : Trigonometry  Operator=cos
  Cos6 : Trigonometry
  Cos8 : Trigonometry
  Degrees to Radians : simulink_extras/Transformations/Degrees to Radians
  Divide{,2..7} (7 alike) : Product  Inputs=*/
  Goto11 : Goto  Commented=on  GotoTag=Pos_M_m
  Integrator : Integrator
  Integrator1 : Integrator
  Integrator2 : Integrator
  Integrator3 : Integrator  InitialCondition=10*pi/180
  Integrator6 : Integrator  InitialCondition=10*pi/180
  Mux : Mux  Inputs=3
  Mux1 : Mux  Inputs=3
  Product{,1..24} (25 alike) : Product
  Scope : Scope
  Scope1 : Scope
  Sin{,3..7,9..10} (8 alike) : Trigonometry
  Sin1 : Trigonometry  Operator=cos
  Sin2 : Trigonometry  Operator=cos
  Sin8 : Trigonometry  Operator=cos
  Sqrt : Sqrt
  Square{,1..4} (5 alike) : Math  Operator=square
  Sum : Sum  Inputs=|+-
  Switch : Switch  Threshold=2  SaturateOnIntegerOverflow=off  InputSameDT=off
  Tan : Trigonometry  Operator=tan
  Tan1 : Trigonometry  Operator=tan
  CMMAV3_state : Outport
  wires:
  [theta_L] -> Tan1/1
  Product16/1 -> Add3/2
  Product9/1 -> Product10/1
  Tan/1 -> Product3/2
  [psi_M] -> Sin9/1
  [theta_M] -> Cos/1
  Sin10/1 -> Product18/2
  [psi_M] -> Sin5/1
  Product17/1 -> Product18/1
  [psi_M] -> Sin10/1
  [V_M_mps] -> Divide/2
  Sin6/1 -> Square1/1
  Product15/1 -> Product16/1
  Cos5/1 -> Product17/2
  Sin/1 -> Square/1
  Add2/1 -> Add3/1
  Divide7/1 -> Product17/1
  [theta_M] -> Sin6/1
  [R] -> Divide7/2
  Sin3/1 -> Product6/2
  Add1/1 -> [theta_M_dot_state]
  Sin9/1 -> Product16/2
  Divide6/1 -> Product15/1
  Square1/1 -> Product15/2
  [R] -> Divide3/2
  [a_z_M] -> Divide/1
  [theta_M] -> Cos5/1
  Add3/1 -> Add4/1
  Product12/1 -> Divide6/2
  Product8/1 -> Product9/1
  [a_y_M] -> Divide4/1
  [psi_M] -> Cos3/1
  Product10/1 -> Product11/1
  Product3/1 -> Product4/1
  Divide4/1 -> Add2/1
  Cos3/1 -> Product10/2
  Product11/1 -> Add2/2
  [R] -> Product12/2
  [V_M_mps] -> Divide5/1
  Cos/1 -> Product4/2
  Product5/1 -> Product6/1
  Product6/1 -> Add1/2
  Divide3/1 -> Product5/1
  Cos1/1 -> Product5/2
  Square/1 -> Product/2
  [psi_M] -> Cos1/1
  [V_M_mps] -> Product7/2
  [R] -> Divide2/2
  [V_M_mps] -> Divide2/1
  [psi_M] -> Sin/1
  [theta_M] -> Sin4/1
  Tan1/1 -> Product11/2
  [theta_M] -> Sin3/1
  Add/1 -> Add1/1
  [R] -> Divide5/2
  [V_M_mps] -> Divide6/1
  Product/1 -> Product3/1
  Add4/1 -> [psi_M_dot_state]
  [V_M_mps] -> Divide7/1
  Cos2/1 -> Product7/1
  Divide2/1 -> Product/1
  [theta_M] -> Cos2/1
  Sin4/1 -> Product8/2
  [theta_L] -> Tan/1
  Cos4/1 -> Product12/1
  [theta_M] -> Cos4/1
  [V_M_mps] -> Divide3/1
  Sin5/1 -> Product9/2
  Product4/1 -> Add/2
  Product18/1 -> Add4/2
  Product7/1 -> Divide4/2
  Divide5/1 -> Product8/1
  Divide/1 -> Add/1
  [V_M_mps] -> Product24/1
  Sin7/1 -> Product24/2
  [V_M_mps] -> Product20/2
  [theta_M] -> Cos11/1
  [psi_M] -> Sin8/1
  Mux1/1 -> Scope1/1, Goto11/1
  [theta_M] -> Sin7/1
  Sin8/1 -> Product14/2
  Product14/1 -> Product19/1
  Product19/1 -> Integrator/1  "X"
  Product13/1 -> Product20/1
  Product24/1 -> Integrator2/1  "Z"
  [psi_M] -> Cos8/1
  [V_M_mps] -> Product19/2
  [theta_M] -> Cos10/1
  Cos11/1 -> Product13/1
  Cos8/1 -> Product13/2
  Product20/1 -> Integrator1/1  "Y"
  Cos10/1 -> Product14/1
  Integrator/1 -> Mux1/1
  Integrator1/1 -> Mux1/2
  Integrator2/1 -> Mux1/3
  CMMAV3_input/1 -> Bus Selector/1
  Integrator3/1 -> [psi_M]
  [theta_M_dot_state] -> Integrator6/1
  [psi_M_dot_state] -> Integrator3/1
  Integrator6/1 -> [theta_M]
  Bus Selector/2 -> [a_y_M]  "<a_y_M>"
  Bus Selector/1 -> [a_z_M]  "<a_z_M>"
  Bus Selector/4 -> [theta_L]  "<theta_L>"
  Bus Selector/3 -> [R]  "<R>"
  Bus Selector/5 -> [psi_L]  "<psi_L>"
  [a_y_M] -> Bus Creator/6
  [Pos_M_m] -> Bus Creator/1  "Pos_M_m"
  [a_z_M] -> Bus Creator/5
  [theta_M] -> Bus Creator/3  "theta_M"
  [psi_M] -> Bus Creator/2  "psi_M"
  Bus Creator/1 -> CMMAV3_state/1
  [V_M_mps] -> Bus Creator/4  "V_M"
  [X] -> Mux/1
  Constant2/1 -> Switch/1
  Sqrt/1 -> Switch/2
  Constant3/1 -> Switch/3
  [Z] -> Square4/1
  Switch/1 -> [V_M_mps]
  Square2/1 -> Add5/1
  Square4/1 -> Add5/3
  Product23/1 -> [Z]  "Z"
  [R] -> Product21/2
  [R] -> Product22/2
  Square3/1 -> Add5/2
  Sum/1 -> Sin1/1
  [theta_L] -> Sum/2
  Add5/1 -> Sqrt/1
  [psi_L] -> Sin2/1
  Degrees to Radians/1 -> Sum/1
  Mux/1 -> [Pos_M_m], Scope/1  "CMMAV3"
  [R] -> Product23/1
  Cos7/1 -> Product2/1
  Sin1/1 -> Product23/2
  [X] -> Square3/1
  [theta_L] -> Cos7/1
  Product1/1 -> Product22/1
  Product2/1 -> Product21/1
  Constant1/1 -> Degrees to Radians/1
  [Z] -> Mux/3
  Sin2/1 -> Product2/2
  Product21/1 -> [X]  "X"
  [Y] -> Mux/2
  [psi_L] -> Cos6/1
  [theta_L] -> Cos9/1
  [Y] -> Square2/1
  Cos9/1 -> Product1/1
  Cos6/1 -> Product1/2
  Product22/1 -> [Y]  "Y"

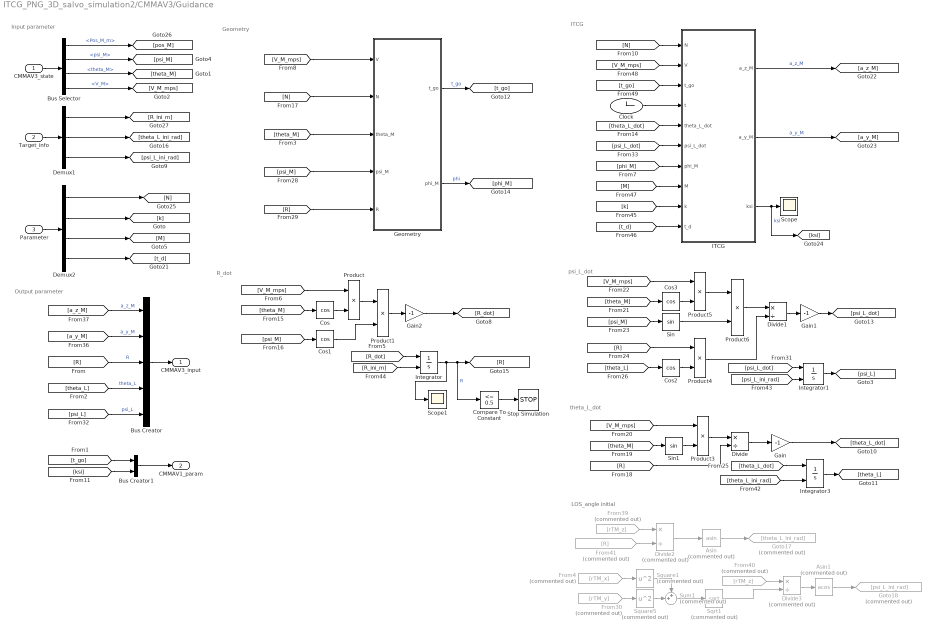
== system ITCG_PNG_3D_salvo_simulation2/CMMAV3/Guidance ==
  note: Input parameter
  note: R_dot
  note: psi_L_dot
  note: theta_L_dot
  note: LOS_angle initial
  note: Output parameter
  note: Geometry
  note: ITCG
  CMMAV3_state : Inport
  Target_info : Inport  Port=2
  Parameter : Inport  Port=3
  Asin : Trigonometry  Commented=on  Operator=asin
  Asin1 : Trigonometry  Commented=on  Operator=acos
  Bus Creator : BusCreator  Inputs=5
  Bus Creator1 : BusCreator  Inputs=2
  Bus Selector : BusSelector  OutputSignals=Pos_M_m,psi_M,theta_M,V_M
  Clock : Clock
  Compare To Constant : simulink/Logic and Bit Operations/Compare To Constant  relop=<=  const=0.5  OutDataTypeStr=boolean
  Cos{,1..3} (4 alike) : Trigonometry  Operator=cos
  Demux1 : Demux  Outputs=3
  Demux2 : Demux
  Divide : Product  Inputs=*/
  Divide1 : Product  Inputs=*/
  Divide2 : Product  Commented=on  Inputs=*/
  Divide3 : Product  Commented=on  Inputs=*/
  From30 : From  Commented=on  GotoTag=rTM_y
  From39 : From  Commented=on  GotoTag=rTM_z
  From4 : From  Commented=on  GotoTag=rTM_x
  From40 : From  Commented=on  GotoTag=rTM_z
  From41 : From  Commented=on  GotoTag=R
  Gain : Gain  Gain=-1
  Gain1 : Gain  Gain=-1
  Gain2 : Gain  Gain=-1
  Geometry : MATLAB Function  TreatAsAtomicUnit=on
  Goto17 : Goto  Commented=on  GotoTag=theta_L_ini_rad
  Goto18 : Goto  Commented=on  GotoTag=psi_L_ini_rad
  ITCG : MATLAB Function  TreatAsAtomicUnit=on
  Integrator : Integrator  InitialConditionSource=external  InitialCondition=sqrt(300^2+500^2+200^2)
  Integrator1 : Integrator  InitialConditionSource=external
  Integrator3 : Integrator  InitialConditionSource=external
  Product{,1,3..6} (6 alike) : Product
  Scope : Scope
  Scope1 : Scope
  Sin : Trigonometry
  Sin1 : Trigonometry
  Sqrt1 : Sqrt  Commented=on
  Square1 : Math  Commented=on  Operator=square
  Square5 : Math  Commented=on  Operator=square
  Stop Simulation : Stop
  Sum1 : Sum  Commented=on  Inputs=++|
  CMMAV3_input : Outport
  CMMAV1_param : Outport  Port=2
  wires:
  Product1/1 -> Gain2/1
  Gain2/1 -> [R_dot]
  [theta_L] -> Cos2/1
  [theta_L_dot] -> Integrator3/1
  Gain/1 -> [theta_L_dot]
  Product5/1 -> Product6/1
  Divide1/1 -> Gain1/1
  [V_M_mps] -> Product3/1
  [V_M_mps] -> Product5/1
  [theta_M] -> Sin1/1
  [R] -> Divide/2
  [theta_M] -> Cos3/1
  Divide/1 -> Gain/1
  [theta_M] -> Cos/1
  [R] -> Product4/1
  Product4/1 -> Divide1/2
  Integrator3/1 -> [theta_L]
  [psi_L_dot] -> Integrator1/1
  Sin1/1 -> Product3/2
  Product3/1 -> Divide/1
  [psi_M] -> Cos1/1
  Cos/1 -> Product/2
  Integrator1/1 -> [psi_L]
  Product6/1 -> Divide1/1
  [psi_M] -> Sin/1
  Compare To Constant/1 -> Stop Simulation/1
  [V_M_mps] -> Product/1
  Cos3/1 -> Product5/2
  Sin/1 -> Product6/2
  Integrator/1 -> Scope1/1, [R], Compare To Constant/1  "R"
  Product/1 -> Product1/1
  Cos2/1 -> Product4/2
  Cos1/1 -> Product1/2
  Gain1/1 -> [psi_L_dot]
  [R_dot] -> Integrator/1
  Divide3/1 -> Asin1/1
  Sum1/1 -> Sqrt1/1
  From30/1 -> Square5/1
  Square5/1 -> Sum1/2
  Square1/1 -> Sum1/1
  Asin/1 -> Goto17/1
  Sqrt1/1 -> Divide3/2
  From41/1 -> Divide2/2
  Asin1/1 -> Goto18/1
  From40/1 -> Divide3/1
  From39/1 -> Divide2/1
  From4/1 -> Square1/1
  Divide2/1 -> Asin/1
  CMMAV3_state/1 -> Bus Selector/1
  Target_info/1 -> Demux1/1
  Demux2/1 -> [N]
  Parameter/1 -> Demux2/1
  Bus Selector/1 -> [pos_M]  "<Pos_M_m>"
  Bus Selector/4 -> [V_M_mps]  "<V_M>"
  Demux1/2 -> [theta_L_ini_rad]
  Demux1/3 -> [psi_L_ini_rad]
  Demux1/1 -> [R_ini_m]
  [psi_L] -> Bus Creator/5  "psi_L"
  [theta_L] -> Bus Creator/4  "theta_L"
  Bus Creator/1 -> CMMAV3_input/1
  [a_y_M] -> Bus Creator/2  "a_y_M"
  [R] -> Bus Creator/3  "R"
  [a_z_M] -> Bus Creator/1  "a_z_M"
  [theta_L_ini_rad] -> Integrator3/2
  [psi_L_ini_rad] -> Integrator1/2
  [R_ini_m] -> Integrator/2
  Bus Selector/2 -> [psi_M]  "<psi_M>"
  Bus Selector/3 -> [theta_M]  "<theta_M>"
  Geometry/1(t_go) -> [t_go]  "t_go"
  [psi_M] -> Geometry/4(psi_M)
  Geometry/2(phi_M) -> [phi_M]  "phi"
  [V_M_mps] -> Geometry/1(V)
  [theta_M] -> Geometry/3(theta_M)
  [R] -> Geometry/5(R)
  [N] -> Geometry/2(N)
  Demux2/2 -> [k]
  Demux2/3 -> [M]
  Demux2/4 -> [t_d]
  [ksi] -> Bus Creator1/2
  [t_go] -> Bus Creator1/1
  Bus Creator1/1 -> CMMAV1_param/1
  ITCG/3(ksi) -> [ksi], Scope/1  "ksi"
  [t_d] -> ITCG/10(t_d)
  ITCG/1(a_z_M) -> [a_z_M]  "a_z_M"
  ITCG/2(a_y_M) -> [a_y_M]  "a_y_M"
  [theta_L_dot] -> ITCG/5(theta_L_dot)
  [phi_M] -> ITCG/7(phi_M)
  [t_go] -> ITCG/3(t_go)
  [N] -> ITCG/1(N)
  [M] -> ITCG/8(M)
  Clock/1 -> ITCG/4(t)
  [V_M_mps] -> ITCG/2(V)
  [k] -> ITCG/9(k)
  [psi_L_dot] -> ITCG/6(psi_L_dot)

== system ITCG_PNG_3D_salvo_simulation2/CMMAV3/Parameter init ==
  Constant : Constant  Value=3
  Constant1 : Constant  Value=2
  Constant2 : Constant  Value=10
  Constant3 : Constant  Value=30
  Mux : Mux
  Parameter : Outport
  wires:
  Mux/1 -> Parameter/1
  Constant3/1 -> Mux/4
  Constant2/1 -> Mux/3
  Constant1/1 -> Mux/2
  Constant/1 -> Mux/1

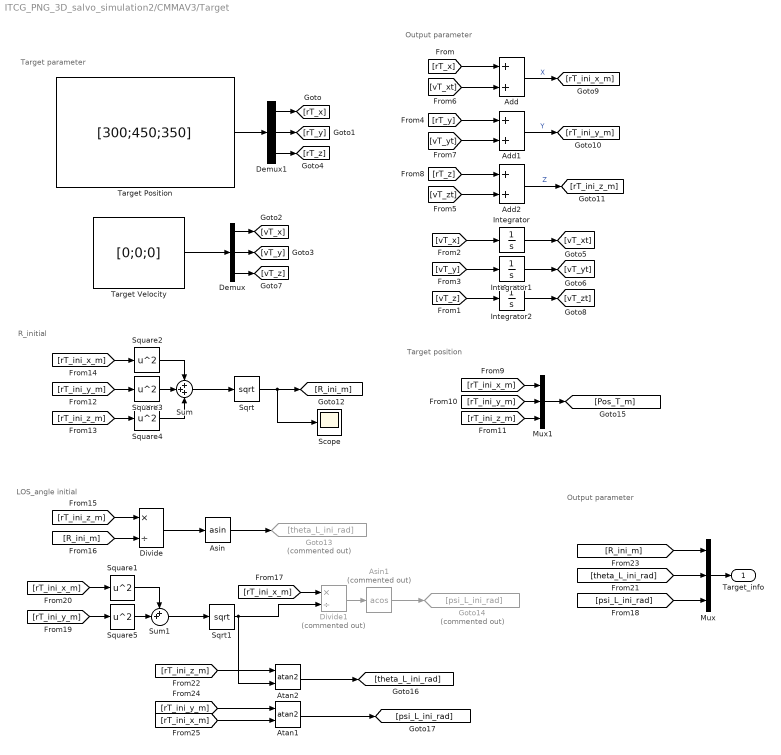
== system ITCG_PNG_3D_salvo_simulation2/CMMAV3/Target ==
  note: LOS_angle initial
  note: Target position
  note: Target parameter
  note: Output parameter
  note: R_initial
  note: Output parameter
  Add : Sum
  Add1 : Sum
  Add2 : Sum
  Asin : Trigonometry  Operator=asin
  Asin1 : Trigonometry  Commented=on  Operator=acos
  Atan1 : Trigonometry  Operator=atan2
  Atan2 : Trigonometry  Operator=atan2
  Demux : Demux  Outputs=3
  Demux1 : Demux  Outputs=3
  Divide : Product  Inputs=*/
  Divide1 : Product  Commented=on  Inputs=*/
  Goto13 : Goto  Commented=on  GotoTag=theta_L_ini_rad
  Goto14 : Goto  Commented=on  GotoTag=psi_L_ini_rad
  Integrator : Integrator
  Integrator1 : Integrator
  Integrator2 : Integrator
  Mux : Mux  Inputs=3
  Mux1 : Mux  Inputs=3
  Scope : Scope
  Sqrt : Sqrt
  Sqrt1 : Sqrt
  Square{1..5} (5 alike) : Math  Operator=square
  Sum : Sum  Inputs=+++
  Sum1 : Sum  Inputs=++|
  Target Position : Constant  Value=[300;450;350]  VectorParams1D=off
  Target Velocity : Constant  Value=[0;0;0]  VectorParams1D=off
  Target_info : Outport
  wires:
  [psi_L_ini_rad] -> Mux/3
  Asin/1 -> Goto13/1
  [rT_ini_z_m] -> Mux1/3
  [rT_z] -> Add2/1
  Demux/3 -> [vT_z]
  [vT_z] -> Integrator2/1
  Demux/2 -> [vT_y]
  [rT_ini_x_m] -> Mux1/1
  Add1/1 -> [rT_ini_y_m]  "Y"
  Square2/1 -> Sum/1
  [vT_x] -> Integrator/1
  Mux1/1 -> [Pos_T_m]
  Square3/1 -> Sum/2
  Add2/1 -> [rT_ini_z_m]  "Z"
  Target Position/1 -> Demux1/1
  Integrator/1 -> [vT_xt]
  Sum/1 -> Sqrt/1
  Demux1/3 -> [rT_z]
  [rT_ini_y_m] -> Mux1/2
  Integrator1/1 -> [vT_yt]
  Demux/1 -> [vT_x]
  Demux1/1 -> [rT_x]
  Target Velocity/1 -> Demux/1
  Demux1/2 -> [rT_y]
  Add/1 -> [rT_ini_x_m]  "X"
  [vT_yt] -> Add1/2
  Divide1/1 -> Asin1/1
  [rT_x] -> Add/1
  [vT_zt] -> Add2/2
  Sum1/1 -> Sqrt1/1
  [rT_ini_x_m] -> Square1/1
  Square1/1 -> Sum1/1
  Square5/1 -> Sum1/2
  [rT_ini_y_m] -> Square5/1
  [vT_y] -> Integrator1/1
  [rT_y] -> Add1/1
  [rT_ini_x_m] -> Square2/1
  [rT_ini_z_m] -> Divide/1
  [R_ini_m] -> Mux/1
  Sqrt/1 -> Scope/1, [R_ini_m]
  [R_ini_m] -> Divide/2
  [rT_ini_z_m] -> Square4/1
  [rT_ini_y_m] -> Square3/1
  [vT_xt] -> Add/2
  Divide/1 -> Asin/1
  Integrator2/1 -> [vT_zt]
  Square4/1 -> Sum/3
  [rT_ini_x_m] -> Divide1/1
  [theta_L_ini_rad] -> Mux/2
  Asin1/1 -> Goto14/1
  Mux/1 -> Target_info/1
  Sqrt1/1 -> Atan2/2, Divide1/2
  [rT_ini_z_m] -> Atan2/1
  Atan2/1 -> [theta_L_ini_rad]
  [rT_ini_x_m] -> Atan1/2
  [rT_ini_y_m] -> Atan1/1
  Atan1/1 -> [psi_L_ini_rad]

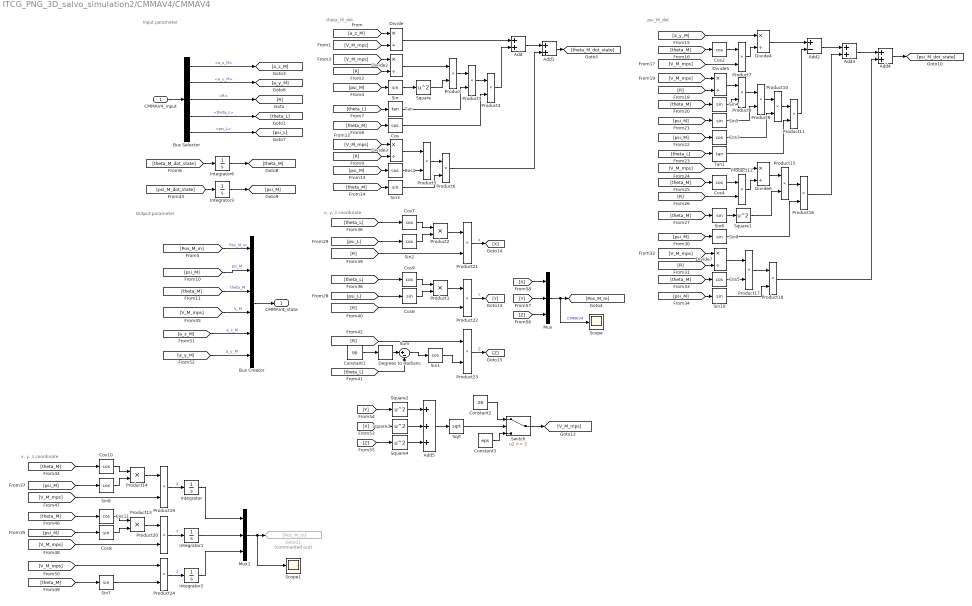
== system ITCG_PNG_3D_salvo_simulation2/CMMAV4/CMMAV4 ==
  note: theta_M_dot
  note: psi_M_dot
  note: x, y, z coordinate
  note: Input parameter
  note: Output parameter
  note: x, y, z coordinate
  CMMAV4_input : Inport
  Add{,1,3..4} (4 alike) : Sum
  Add2 : Sum  Inputs=+-
  Add5 : Sum  Inputs=+++
  Bus Creator : BusCreator  Inputs=6
  Bus Selector : BusSelector  OutputSignals=a_z_M,a_y_M,R,theta_L,psi_L
  Constant1 : Constant  Value=90
  Constant2 : Constant  Value=28
  Constant3 : Constant  Value=eps
  Cos{,1..5,7,9..11} (10 alike) : Trigonometry  Operator=cos
  Cos6 : Trigonometry
  Cos8 : Trigonometry
  Degrees to Radians : simulink_extras/Transformations/Degrees to Radians
  Divide{,2..7} (7 alike) : Product  Inputs=*/
  Goto11 : Goto  Commented=on  GotoTag=Pos_M_m
  Integrator : Integrator
  Integrator1 : Integrator
  Integrator2 : Integrator
  Integrator3 : Integrator  InitialCondition=10*pi/180
  Integrator6 : Integrator  InitialCondition=10*pi/180
  Mux : Mux  Inputs=3
  Mux1 : Mux  Inputs=3
  Product{,1..24} (25 alike) : Product
  Scope : Scope
  Scope1 : Scope
  Sin{,3..7,9..10} (8 alike) : Trigonometry
  Sin1 : Trigonometry  Operator=cos
  Sin2 : Trigonometry  Operator=cos
  Sin8 : Trigonometry  Operator=cos
  Sqrt : Sqrt
  Square{,1..4} (5 alike) : Math  Operator=square
  Sum : Sum  Inputs=|+-
  Switch : Switch  Threshold=2  SaturateOnIntegerOverflow=off  InputSameDT=off
  Tan : Trigonometry  Operator=tan
  Tan1 : Trigonometry  Operator=tan
  CMMAV4_state : Outport
  wires:
  [theta_L] -> Tan1/1
  Product16/1 -> Add3/2
  Product9/1 -> Product10/1
  Tan/1 -> Product3/2
  [psi_M] -> Sin9/1
  [theta_M] -> Cos/1
  Sin10/1 -> Product18/2
  [psi_M] -> Sin5/1
  Product17/1 -> Product18/1
  [psi_M] -> Sin10/1
  [V_M_mps] -> Divide/2
  Sin6/1 -> Square1/1
  Product15/1 -> Product16/1
  Cos5/1 -> Product17/2
  Sin/1 -> Square/1
  Add2/1 -> Add3/1
  Divide7/1 -> Product17/1
  [theta_M] -> Sin6/1
  [R] -> Divide7/2
  Sin3/1 -> Product6/2
  Add1/1 -> [theta_M_dot_state]
  Sin9/1 -> Product16/2
  Divide6/1 -> Product15/1
  Square1/1 -> Product15/2
  [R] -> Divide3/2
  [a_z_M] -> Divide/1
  [theta_M] -> Cos5/1
  Add3/1 -> Add4/1
  Product12/1 -> Divide6/2
  Product8/1 -> Product9/1
  [a_y_M] -> Divide4/1
  [psi_M] -> Cos3/1
  Product10/1 -> Product11/1
  Product3/1 -> Product4/1
  Divide4/1 -> Add2/1
  Cos3/1 -> Product10/2
  Product11/1 -> Add2/2
  [R] -> Product12/2
  [V_M_mps] -> Divide5/1
  Cos/1 -> Product4/2
  Product5/1 -> Product6/1
  Product6/1 -> Add1/2
  Divide3/1 -> Product5/1
  Cos1/1 -> Product5/2
  Square/1 -> Product/2
  [psi_M] -> Cos1/1
  [V_M_mps] -> Product7/2
  [R] -> Divide2/2
  [V_M_mps] -> Divide2/1
  [psi_M] -> Sin/1
  [theta_M] -> Sin4/1
  Tan1/1 -> Product11/2
  [theta_M] -> Sin3/1
  Add/1 -> Add1/1
  [R] -> Divide5/2
  [V_M_mps] -> Divide6/1
  Product/1 -> Product3/1
  Add4/1 -> [psi_M_dot_state]
  [V_M_mps] -> Divide7/1
  Cos2/1 -> Product7/1
  Divide2/1 -> Product/1
  [theta_M] -> Cos2/1
  Sin4/1 -> Product8/2
  [theta_L] -> Tan/1
  Cos4/1 -> Product12/1
  [theta_M] -> Cos4/1
  [V_M_mps] -> Divide3/1
  Sin5/1 -> Product9/2
  Product4/1 -> Add/2
  Product18/1 -> Add4/2
  Product7/1 -> Divide4/2
  Divide5/1 -> Product8/1
  Divide/1 -> Add/1
  [V_M_mps] -> Product24/1
  Sin7/1 -> Product24/2
  [V_M_mps] -> Product20/2
  [theta_M] -> Cos11/1
  [psi_M] -> Sin8/1
  Mux1/1 -> Scope1/1, Goto11/1
  [theta_M] -> Sin7/1
  Sin8/1 -> Product14/2
  Product14/1 -> Product19/1
  Product19/1 -> Integrator/1  "X"
  Product13/1 -> Product20/1
  Product24/1 -> Integrator2/1  "Z"
  [psi_M] -> Cos8/1
  [V_M_mps] -> Product19/2
  [theta_M] -> Cos10/1
  Cos11/1 -> Product13/1
  Cos8/1 -> Product13/2
  Product20/1 -> Integrator1/1  "Y"
  Cos10/1 -> Product14/1
  Integrator/1 -> Mux1/1
  Integrator1/1 -> Mux1/2
  Integrator2/1 -> Mux1/3
  CMMAV4_input/1 -> Bus Selector/1
  Integrator3/1 -> [psi_M]
  [theta_M_dot_state] -> Integrator6/1
  [psi_M_dot_state] -> Integrator3/1
  Integrator6/1 -> [theta_M]
  Bus Selector/2 -> [a_y_M]  "<a_y_M>"
  Bus Selector/1 -> [a_z_M]  "<a_z_M>"
  Bus Selector/4 -> [theta_L]  "<theta_L>"
  Bus Selector/3 -> [R]  "<R>"
  Bus Selector/5 -> [psi_L]  "<psi_L>"
  [a_y_M] -> Bus Creator/6  "a_y_M"
  [Pos_M_m] -> Bus Creator/1  "Pos_M_m"
  [a_z_M] -> Bus Creator/5  "a_z_M"
  [theta_M] -> Bus Creator/3  "theta_M"
  [psi_M] -> Bus Creator/2  "psi_M"
  Bus Creator/1 -> CMMAV4_state/1
  [V_M_mps] -> Bus Creator/4  "V_M"
  [X] -> Mux/1
  Constant2/1 -> Switch/1
  Sqrt/1 -> Switch/2
  Constant3/1 -> Switch/3
  [Z] -> Square4/1
  Switch/1 -> [V_M_mps]
  Square2/1 -> Add5/1
  Square4/1 -> Add5/3
  Product23/1 -> [Z]  "Z"
  [R] -> Product21/2
  [R] -> Product22/2
  Square3/1 -> Add5/2
  Sum/1 -> Sin1/1
  [theta_L] -> Sum/2
  Add5/1 -> Sqrt/1
  [psi_L] -> Sin2/1
  Degrees to Radians/1 -> Sum/1
  Mux/1 -> [Pos_M_m], Scope/1  "CMMAV4"
  [R] -> Product23/1
  Cos7/1 -> Product2/1
  Sin1/1 -> Product23/2
  [X] -> Square3/1
  [theta_L] -> Cos7/1
  Product1/1 -> Product22/1
  Product2/1 -> Product21/1
  Constant1/1 -> Degrees to Radians/1
  [Z] -> Mux/3
  Sin2/1 -> Product2/2
  Product21/1 -> [X]  "X"
  [Y] -> Mux/2
  [psi_L] -> Cos6/1
  [theta_L] -> Cos9/1
  [Y] -> Square2/1
  Cos9/1 -> Product1/1
  Cos6/1 -> Product1/2
  Product22/1 -> [Y]  "Y"
